simulink model "pemfc_aekf"  (R2024a)
settings: Solver=FixedStepDiscrete  StartTime=0.0  StopTime=10.0  RelTol=1e-3
values from neighbouring files (symbols this model uses):
  Ts = u(9)    [pemfc_step_paper_clean.m]
libraries: sharedTrackingLibrary x1
settings Model: Creator=belit  LastModifiedBy=belit

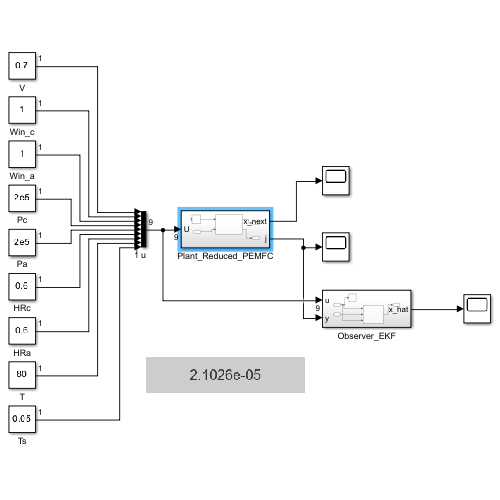
[thumbnail: Simulink's stored preview of the top-level diagram]
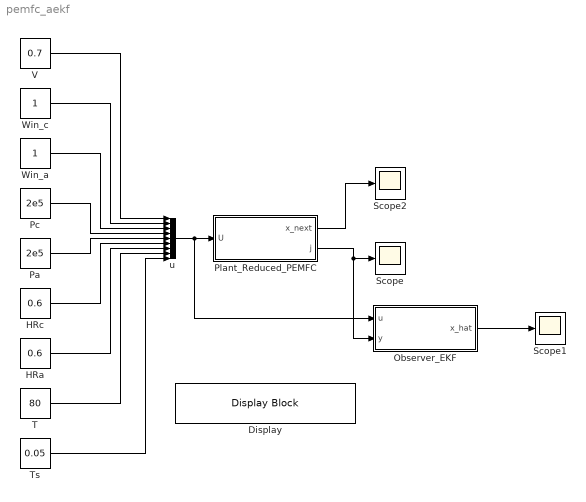
== system pemfc_aekf ==
  Display : DisplayBlock  LabelPosition=Hide  Transparency=1
  HRa : Constant  Value=0.6
  HRc : Constant  Value=0.6
  Observer_EKF : Subsystem
  Pa : Constant  Value=2e5
  Pc : Constant  Value=2e5
  Plant_Reduced_PEMFC : Subsystem
  Scope : Scope
  Scope1 : Scope
  Scope2 : Scope
  T : Constant  Value=80  SampleTime=Ts
  Ts : Constant  Value=0.05
  V : Constant  Value=0.7
  Win_a : Constant
  Win_c : Constant
  u : Mux  Inputs=9
  wires:
  V/1 -> u/1
  Win_c/1 -> u/2
  Win_a/1 -> u/3
  Pc/1 -> u/4
  Pa/1 -> u/5
  HRc/1 -> u/6
  HRa/1 -> u/7
  T/1 -> u/8
  u/1 -> Plant_Reduced_PEMFC/1(U), Observer_EKF/1(u)
  Plant_Reduced_PEMFC/2(j) -> Scope/1, Observer_EKF/2(y)
  Observer_EKF/1(x_hat) -> Scope1/1
  Ts/1 -> u/9
  Plant_Reduced_PEMFC/1(x_next) -> Scope2/1

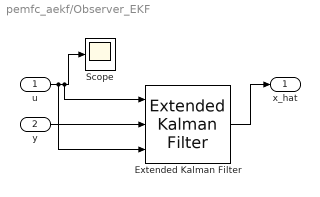
== system pemfc_aekf/Observer_EKF ==
  u : Inport
  y : Inport  Port=2
  Extended Kalman Filter : sharedTrackingLibrary/Extended Kalman Filter  StateTransitionFcn=f_stub  HasStateTransitionJacobianFcn=off  HasAdditiveProcessNoise=Additive  ProcessNoise=1e-4*eye(3)  HasTimeVaryingProcessNoise=off  HasStateTransitionFcnExtraArgument=1  InitialState=[10;10;10]  InitialStateCovariance=eye(3)  MeasurementFcn1=h_stub  HasMeasurementJacobianFcn1=off  HasMeasurementEnablePort1=off  HasAdditiveMeasurementNoise1=Additive  MeasurementNoise1=1e-2  HasTimeVaryingMeasurementNoise1=off  HasMeasurementFcnExtraArgument1=1  HasMeasurementWrapping1=off  MeasurementFcn2=myMeasurementFcn  HasMeasurementJacobianFcn2=off  HasMeasurementEnablePort2=off  HasAdditiveMeasurementNoise2=Additive  MeasurementNoise2=1  HasTimeVaryingMeasurementNoise2=off  HasMeasurementFcnExtraArgument2=0  HasMeasurementWrapping2=off  MeasurementFcn3=myMeasurementFcn  HasMeasurementJacobianFcn3=off  HasMeasurementEnablePort3=off  HasAdditiveMeasurementNoise3=Additive  MeasurementNoise3=1  HasTimeVaryingMeasurementNoise3=off  HasMeasurementFcnExtraArgument3=0  HasMeasurementWrapping3=off  MeasurementFcn4=myMeasurementFcn  HasMeasurementJacobianFcn4=off  HasMeasurementEnablePort4=off  HasAdditiveMeasurementNoise4=Additive  MeasurementNoise4=1  HasTimeVaryingMeasurementNoise4=off  HasMeasurementFcnExtraArgument4=0  HasMeasurementWrapping4=off  MeasurementFcn5=myMeasurementFcn  HasMeasurementJacobianFcn5=off  HasMeasurementEnablePort5=off  HasAdditiveMeasurementNoise5=Additive  MeasurementNoise5=1  HasTimeVaryingMeasurementNoise5=off  HasMeasurementFcnExtraArgument5=0  HasMeasurementWrapping5=off  EnableMultirate=off  StateTransitionFcnSampleTime=1  MeasurementFcn1SampleTime=1  MeasurementFcn2SampleTime=1  MeasurementFcn3SampleTime=1  MeasurementFcn4SampleTime=1  MeasurementFcn5SampleTime=1  UseCurrentEstimator=on  OutputStateCovariance=off  DataType=double  SampleTime=Ts  NumberOfMeasurements=1
  Scope : Scope
  x_hat : Outport
  wires:
  y/1 -> Extended Kalman Filter/2
  Extended Kalman Filter/1 -> x_hat/1
  u/1 -> Extended Kalman Filter/3, Extended Kalman Filter/1, Scope/1

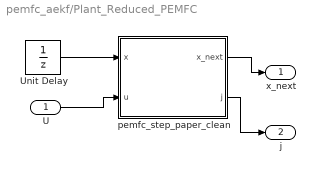
== system pemfc_aekf/Plant_Reduced_PEMFC ==
  U : Inport
  Unit Delay : UnitDelay  InitialCondition=[10;10;10]  SampleTime=Ts  HasFrameUpgradeWarning=on
  pemfc_step_paper_clean : MATLAB Function  TreatAsAtomicUnit=on
  x_next : Outport
  j : Outport  Port=2
  wires:
  pemfc_step_paper_clean/1(x_next) -> x_next/1
  pemfc_step_paper_clean/2(j) -> j/1
  Unit Delay/1 -> pemfc_step_paper_clean/1(x)
  U/1 -> pemfc_step_paper_clean/2(u)

== matlab function pemfc_aekf/Plant_Reduced_PEMFC/pemfc_step_paper_clean ==
  data: x input; u input; x_next output; j output
function [x_next, j] = pemfc_step_stub(x, u)
%#codegen
[x_next, j] = pemfc_step_paper_clean(x, u);
end
